simulink model "sys_ctrl_obs_kalman_lineal_int_theta"  (Simulink 7.9)
settings: Solver=ode45  StartTime=0.0  StopTime=Tt  RelTol=1e-3
undefined symbols (not defined in the file): Ad, Bd, Cd, Dd, K, Knoise, P0, Qd, Rd, Ts, x_0
settings Model: Creator=pdoren  LastModifiedBy=matias  CovModelRefEnable=off
settings SolverCC: ZeroCrossAlgorithm=Adaptive
settings DataIOCC: SaveFormat=StructureWithTime  SignalLoggingSaveFormat=Dataset
settings OptimizationCC: ExpressionDepthLimit=128
settings DebuggingCC: UnderspecifiedInitializationDetection=Simplified  MergeDetectMultiDrivingBlocksExec=error  SolverPrmCheckMsg=none  StateNameClashWarn=none
settings HardwareCC: ProdBitPerPointer=64  ProdLargestAtomicFloat=Float  ProdIntDivRoundTo=Zero  ProdEndianess=LittleEndian  ProdHWDeviceType=Specified
settings CodeAppCC: CustomSymbolStrType=$N$R$M_T
settings GRTTargetCC: CodeReplacementLibrary=C89/C90 (ANSI)  GeneratePreprocessorConditionals=Use local settings  CombineOutputUpdateFcns=off  GRTInterface=on

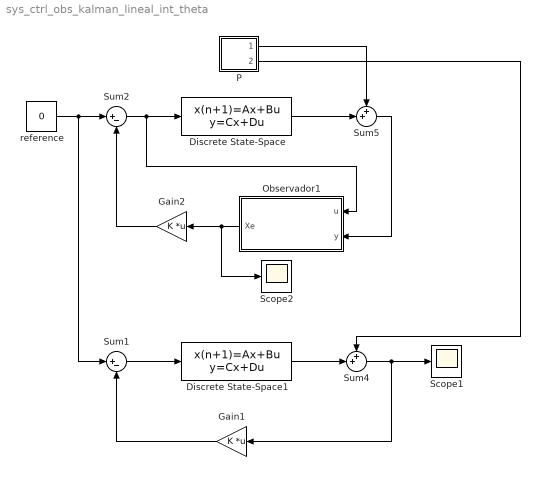
== system sys_ctrl_obs_kalman_lineal_int_theta ==
  Discrete State-Space : DiscreteStateSpace  A=Ad  B=Bd  C=Cd  D=Dd  X0=x_0  SampleTime=Ts
  Discrete State-Space1 : DiscreteStateSpace  A=Ad  B=Bd  C=eye(5)  D=zeros(5,1)  X0=x_0  SampleTime=Ts
  Gain1 : Gain  Gain=K  Multiplication=Matrix(K*u)
  Gain2 : Gain  Gain=K  Multiplication=Matrix(K*u)
  Observador1 : Subsystem
  P : Subsystem
  Scope1 : Scope
      settings: YMin=-2.0207  YMax=4.74305  SaveName=states_lineal_d
  Scope2 : Scope
      settings: YMin=-1246404085495577300000000000000000000000000000000000000000000000000000000000000000000000000000000000000000000000000000000000000000000000000000000000000000000000000000000000000000000000000000000000000000000000000000000000000000000000000000000000000000000000000000000000000000000000000000000000000000000000000.00000  YMax=4973481579999159400000000000000000000000000000000000000000000000000000000000000000000000000000000000000000000000000000000000000000000000000000000000000000000000000000000000000000000000000000000000000000000000000000000000000000000000000000000000000000000000000000000000000000000000000000000000000000000000000.00000  SaveName=states_lineal_d_obs
  Sum1 : Sum  Inputs=|+-
  Sum2 : Sum  Inputs=|+-
  Sum4 : Sum  Inputs=++|
  Sum5 : Sum  Inputs=++|
  reference : Constant  Value=0
  wires:
  Sum2/1 -> Discrete State-Space/1, Observador1/1(u)
  Gain2/1 -> Sum2/2
  Discrete State-Space/1 -> Sum5/2
  reference/1 -> Sum1/1, Sum2/1
  Sum1/1 -> Discrete State-Space1/1
  Gain1/1 -> Sum1/2
  Discrete State-Space1/1 -> Sum4/2
  Sum4/1 -> Gain1/1, Scope1/1
  P/2(Noise5) -> Sum4/1
  P/1(Noise3) -> Sum5/1
  Observador1/1(Xe) -> Gain2/1, Scope2/1
  Sum5/1 -> Observador1/2(y)

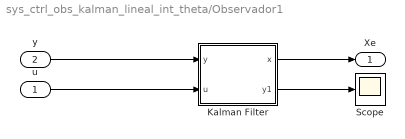
== system sys_ctrl_obs_kalman_lineal_int_theta/Observador1 ==
  u : Inport
  y : Inport  Port=2
  Kalman Filter : Subsystem  mask{x0=0, P0=P0, A=Ad, B=Bd, C=Cd, D=Dd, Q=Qd, R=Rd}
      mask help:
      | Linear Random Process
      | x(k+1)=Ax(k)+Bu(k)+w
      | y(k)=Cx(k)+Du(k)+v
      | w~N(0,Q)
      | w~N(0,R)
      mask Display:
      | disp(sprintf('Kalman\n Filter'))
      | port_label('output',2,'y')
      | port_label('output',1,'x')
      | port_label('input',1,'y')
      | port_label('input',2,'u')
  Scope : Scope
      settings: YMin=-10  YMax=10
  Xe : Outport
  wires:
  Kalman Filter/1(x) -> Xe/1
  Kalman Filter/2(y1) -> Scope/1
  y/1 -> Kalman Filter/1(y)
  u/1 -> Kalman Filter/2(u)

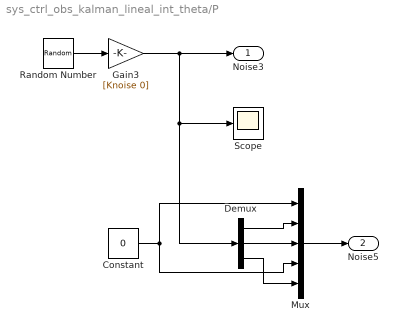
== system sys_ctrl_obs_kalman_lineal_int_theta/P ==
  Constant : Constant  Value=0
  Demux : Demux  Outputs=3
  Gain3 : Gain  Gain=[Knoise 0]
  Mux : Mux  Inputs=5
  Random Number : RandomNumber  SampleTime=Ts
  Scope : Scope
      settings: YMin=-1.00000  YMax=1.00000
  Noise3 : Outport
  Noise5 : Outport  Port=2
  wires:
  Random Number/1 -> Gain3/1
  Gain3/1 -> Noise3/1, Demux/1, Scope/1
  Mux/1 -> Noise5/1
  Demux/1 -> Mux/2
  Demux/2 -> Mux/3
  Constant/1 -> Mux/4, Mux/1
  Demux/3 -> Mux/5

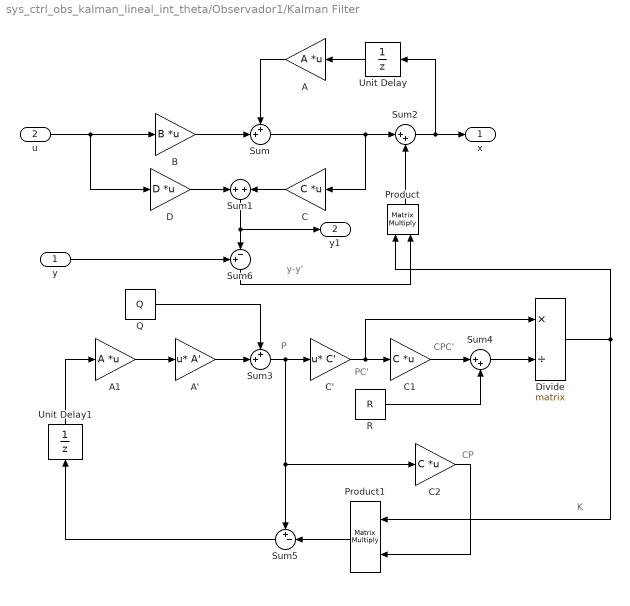
== system sys_ctrl_obs_kalman_lineal_int_theta/Observador1/Kalman Filter ==
  note: P
  note: PC'
  note: CPC'
  note: K
  note: CP
  note: y-y'
  y : Inport
  u : Inport  Port=2  PortDimensions=size(B,2)
  A : Gain  Gain=A  Multiplication=Matrix(K*u)
  A' : Gain  Gain=A'  Multiplication=Matrix(u*K)
  A1 : Gain  Gain=A  Multiplication=Matrix(K*u)
  B : Gain  Gain=B  Multiplication=Matrix(K*u)
  C : Gain  Gain=C  Multiplication=Matrix(K*u)
  C' : Gain  Gain=C'  Multiplication=Matrix(u*K)
  C1 : Gain  Gain=C  Multiplication=Matrix(K*u)
  C2 : Gain  Gain=C  Multiplication=Matrix(K*u)
  D : Gain  Gain=D  Multiplication=Matrix(K*u)
  Divide : Product  Inputs=*/  Multiplication=Matrix(*)
  Product : Product  Multiplication=Matrix(*)  RndMeth=Zero
  Product1 : Product  Multiplication=Matrix(*)  RndMeth=Zero
  Q : Constant  Value=Q
  R : Constant  Value=R
  Sum : Sum  Inputs=++|
  Sum1 : Sum  Inputs=+|+
  Sum2 : Sum  Inputs=|++
  Sum3 : Sum  Inputs=++|
  Sum4 : Sum  Inputs=|++
  Sum5 : Sum  Inputs=+-|
  Sum6 : Sum  Inputs=+-|
  Unit Delay : UnitDelay  X0=x0  SampleTime=Ts
  Unit Delay1 : UnitDelay  X0=P0  SampleTime=Ts
  x : Outport
  y1 : Outport  Port=2
  wires:
  u/1 -> B/1, D/1
  B/1 -> Sum/2
  A/1 -> Sum/1
  Unit Delay/1 -> A/1
  Sum/1 -> Sum2/1, C/1
  Sum2/1 -> x/1, Unit Delay/1
  D/1 -> Sum1/1
  C/1 -> Sum1/2
  A1/1 -> A'/1
  A'/1 -> Sum3/2
  Q/1 -> Sum3/1
  Sum3/1 -> C'/1, Sum5/1, C2/1
  C'/1 -> C1/1, Divide/1
  Product/1 -> Sum2/2
  Divide/1 -> Product/1, Product1/1
  Product1/1 -> Sum5/2
  C1/1 -> Sum4/1
  R/1 -> Sum4/2
  Sum4/1 -> Divide/2
  Unit Delay1/1 -> A1/1
  Sum5/1 -> Unit Delay1/1
  C2/1 -> Product1/2
  Sum1/1 -> Sum6/2, y1/1
  y/1 -> Sum6/1
  Sum6/1 -> Product/2
